simulink model "starter_model"  (R2026a)
settings: Solver=FixedStepDiscrete  StopTime=inf  FixedStep=0.01  EnableMultiTasking=on
undefined symbols (not defined in the file): dspblkCoreblockFVToolHelper, gcbh
settings Model: SILPILModeSetting=veronly  ExtModeTrigDuration=2  Creator=AdePratamaSuryoKusum  LastModifiedBy=AdePratamaSuryoKusum
settings DataIOCC: ExternalInput=milInput
settings HardwareCC: ProdBitPerInt=16.0  ProdBitPerPointer=16.0  ProdBitPerSizeT=16.0  ProdBitPerPtrDiffT=16.0  ProdWordSize=8.0  ProdHWDeviceType=Atmel->AVR
settings RTWCC: SystemTargetFile=ert.tlc  HardwareBoard=Arduino Uno  TLCOptions="-aInlineSetEventsForThisBaseRateFcn=TLC_FALSE -aSuppressMultiTaskScheduler=TLC_FALSE   -aRateBasedStepFcn=1"  Toolchain=Arduino AVR  BuildConfiguration=Faster Runs  Description=Embedded Coder
settings ERTTargetCC: ExtModeTransport=3.0  ExtModeAutomaticAllocSize=off  ExtModeStaticAllocSize=250.0  SupportContinuousTime=on  SupportVariableSizeSignals=on

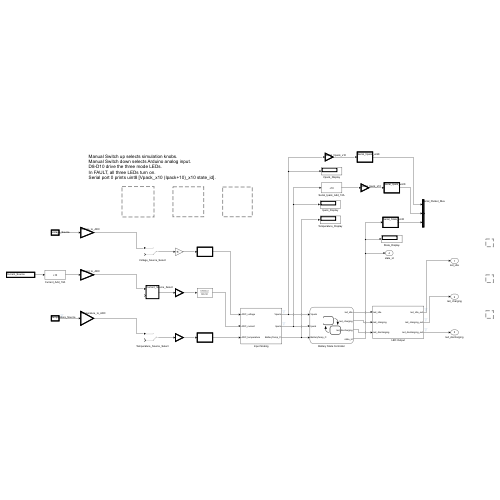
[thumbnail: Simulink's stored preview of the top-level diagram]
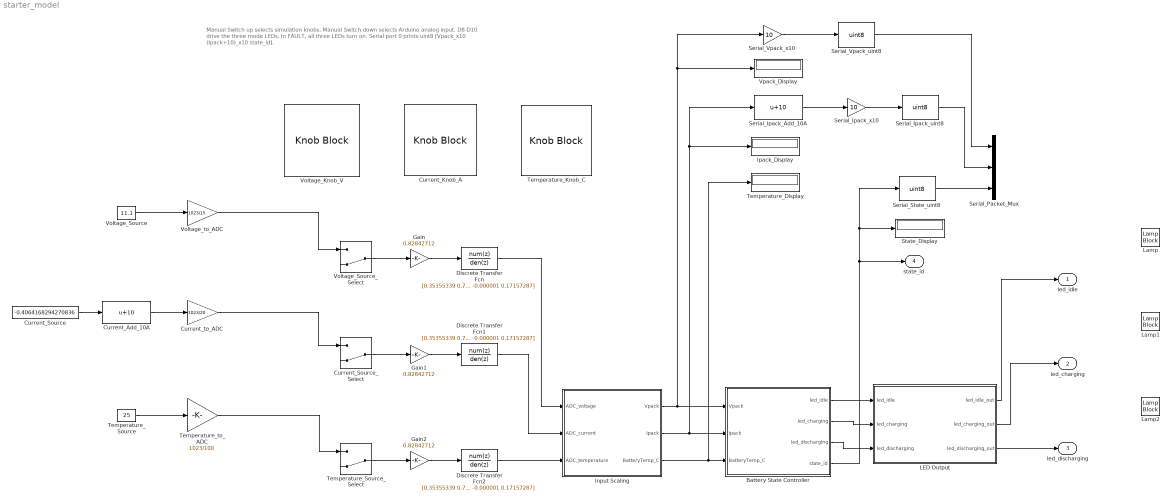
== system starter_model ==
  note: Manual Switch up selects simulation knobs.
      | Manual Switch down selects Arduino analog input.
      | D8-D10 drive the three mode LEDs.
      | In FAULT, all three LEDs turn on.
      | Serial port 0 prints uint8 [Vpack_x10 (Ipack+10)_x10 state_id].
  Battery State Controller : Stateflow chart  TreatAsAtomicUnit=on
  Current_Add_10A : Bias  Bias=10  SaturateOnIntegerOverflow=off
  Current_Knob_A : KnobBlock  ScaleMin=-10  ScaleMax=10
  Current_Source : Constant  Value=-0.4064168294270836
  Current_Source_Select : ManualSwitch  CurrentSetting=0
  Current_to_ADC : Gain  Gain=1023/20
  Discrete Transfer Fcn : DiscreteTransferFcn  LoadFcn=dspblkCoreblockFVToolHelper(gcbh,'load');  Numerator=[0.35355339 0.70710678 0.35355339]  Denominator=[1 -0.000001 0.17157287]
      settings: CopyFcn=dspblkCoreblockFVToolHelper(gcbh,'copy');  DeleteFcn=dspblkCoreblockFVToolHelper(gcbh,'close');  ModelCloseFcn=dspblkCoreblockFVToolHelper(gcbh,'close');  PreSaveFcn=dspblkCoreblockFVToolHelper(gcbh,'presave');  PostSaveFcn=dspblkCoreblockFVToolHelper(gcbh,'postsave');  CloseFcn=dspblkCoreblockFVToolHelper(gcbh,'close');
  Discrete Transfer Fcn1 : DiscreteTransferFcn  LoadFcn=dspblkCoreblockFVToolHelper(gcbh,'load');  Numerator=[0.35355339 0.70710678 0.35355339]  Denominator=[1 -0.000001 0.17157287]
      settings: CopyFcn=dspblkCoreblockFVToolHelper(gcbh,'copy');  DeleteFcn=dspblkCoreblockFVToolHelper(gcbh,'close');  ModelCloseFcn=dspblkCoreblockFVToolHelper(gcbh,'close');  PreSaveFcn=dspblkCoreblockFVToolHelper(gcbh,'presave');  PostSaveFcn=dspblkCoreblockFVToolHelper(gcbh,'postsave');  CloseFcn=dspblkCoreblockFVToolHelper(gcbh,'close');
  Discrete Transfer Fcn2 : DiscreteTransferFcn  LoadFcn=dspblkCoreblockFVToolHelper(gcbh,'load');  Numerator=[0.35355339 0.70710678 0.35355339]  Denominator=[1 -0.000001 0.17157287]
      settings: CopyFcn=dspblkCoreblockFVToolHelper(gcbh,'copy');  DeleteFcn=dspblkCoreblockFVToolHelper(gcbh,'close');  ModelCloseFcn=dspblkCoreblockFVToolHelper(gcbh,'close');  PreSaveFcn=dspblkCoreblockFVToolHelper(gcbh,'presave');  PostSaveFcn=dspblkCoreblockFVToolHelper(gcbh,'postsave');  CloseFcn=dspblkCoreblockFVToolHelper(gcbh,'close');
  Gain : Gain  Gain=0.82842712
  Gain1 : Gain  Gain=0.82842712
  Gain2 : Gain  Gain=0.82842712
  Input Scaling : Subsystem
  Ipack_Display : Display
  LED Output : Subsystem
  Lamp : LampBlock  LabelPosition=Hide  DefaultColor=[192.0, 192.0, 192.0]
  Lamp1 : LampBlock  LabelPosition=Hide  DefaultColor=[192.0, 192.0, 192.0]
  Lamp2 : LampBlock  LabelPosition=Hide  DefaultColor=[192.0, 192.0, 192.0]
  Serial_Ipack_Add_10A : Bias  Bias=10  SaturateOnIntegerOverflow=off
  Serial_Ipack_uint8 : DataTypeConversion  OutDataTypeStr=uint8  SaturateOnIntegerOverflow=off  RndMeth=Floor
  Serial_Ipack_x10 : Gain  Gain=10
  Serial_Packet_Mux : Mux  Inputs=3
  Serial_State_uint8 : DataTypeConversion  OutDataTypeStr=uint8  SaturateOnIntegerOverflow=off  RndMeth=Floor
  Serial_Vpack_uint8 : DataTypeConversion  OutDataTypeStr=uint8  SaturateOnIntegerOverflow=off  RndMeth=Floor
  Serial_Vpack_x10 : Gain  Gain=10
  State_Display : Display
  Temperature_Display : Display
  Temperature_Knob_C : KnobBlock
  Temperature_Source : Constant  Value=25
  Temperature_Source_Select : ManualSwitch  CurrentSetting=0
  Temperature_to_ADC : Gain  Gain=1023/100
  Voltage_Knob_V : KnobBlock  ScaleMax=15
  Voltage_Source : Constant  Value=11.1
  Voltage_Source_Select : ManualSwitch  CurrentSetting=0
  Voltage_to_ADC : Gain  Gain=1023/15
  Vpack_Display : Display
  led_idle : Outport
  led_charging : Outport  Port=2
  led_discharging : Outport  Port=3
  state_id : Outport  Port=4
  wires:
  Current_Add_10A/1 -> Current_to_ADC/1
  Current_Source/1 -> Current_Add_10A/1
  Input Scaling/1(Vpack) -> Battery State Controller/1(Vpack), Serial_Vpack_x10/1, Vpack_Display/1
  Voltage_to_ADC/1 -> Voltage_Source_Select/1
  Voltage_Source_Select/1 -> Gain/1
  Voltage_Source/1 -> Voltage_to_ADC/1
  Temperature_Source_Select/1 -> Gain2/1
  Temperature_Source/1 -> Temperature_to_ADC/1
  Current_to_ADC/1 -> Current_Source_Select/1
  Temperature_to_ADC/1 -> Temperature_Source_Select/1
  Current_Source_Select/1 -> Gain1/1
  Input Scaling/2(Ipack) -> Ipack_Display/1, Serial_Ipack_Add_10A/1, Battery State Controller/2(Ipack)
  Input Scaling/3(BatteryTemp_C) -> Temperature_Display/1, Battery State Controller/3(BatteryTemp_C)
  Serial_Vpack_x10/1 -> Serial_Vpack_uint8/1
  Serial_Ipack_Add_10A/1 -> Serial_Ipack_x10/1
  Battery State Controller/1(led_idle) -> LED Output/1(led_idle)
  LED Output/2(led_charging_out) -> led_charging/1
  Battery State Controller/2(led_charging) -> LED Output/2(led_charging)
  Battery State Controller/3(led_discharging) -> LED Output/3(led_discharging)
  Battery State Controller/4(state_id) -> Serial_State_uint8/1, State_Display/1, state_id/1
  Serial_Vpack_uint8/1 -> Serial_Packet_Mux/1
  Serial_State_uint8/1 -> Serial_Packet_Mux/3
  Serial_Ipack_x10/1 -> Serial_Ipack_uint8/1
  LED Output/1(led_idle_out) -> led_idle/1
  LED Output/3(led_discharging_out) -> led_discharging/1
  Serial_Ipack_uint8/1 -> Serial_Packet_Mux/2
  Discrete Transfer Fcn/1 -> Input Scaling/1(ADC_voltage)
  Discrete Transfer Fcn1/1 -> Input Scaling/2(ADC_current)
  Discrete Transfer Fcn2/1 -> Input Scaling/3(ADC_temperature)
  Gain/1 -> Discrete Transfer Fcn/1
  Gain1/1 -> Discrete Transfer Fcn1/1
  Gain2/1 -> Discrete Transfer Fcn2/1

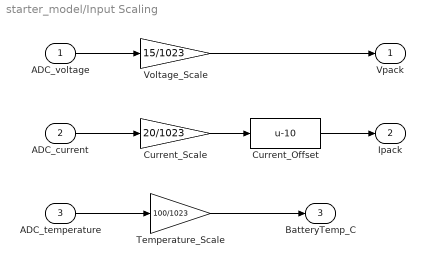
== system starter_model/Input Scaling ==
  ADC_voltage : Inport
  ADC_current : Inport  Port=2
  ADC_temperature : Inport  Port=3
  Current_Offset : Bias  Bias=-10  SaturateOnIntegerOverflow=off
  Current_Scale : Gain  Gain=20/1023
  Temperature_Scale : Gain  Gain=100/1023
  Voltage_Scale : Gain  Gain=15/1023
  Vpack : Outport
  Ipack : Outport  Port=2
  BatteryTemp_C : Outport  Port=3
  wires:
  ADC_voltage/1 -> Voltage_Scale/1
  Voltage_Scale/1 -> Vpack/1
  ADC_current/1 -> Current_Scale/1
  Current_Scale/1 -> Current_Offset/1
  Current_Offset/1 -> Ipack/1
  ADC_temperature/1 -> Temperature_Scale/1
  Temperature_Scale/1 -> BatteryTemp_C/1

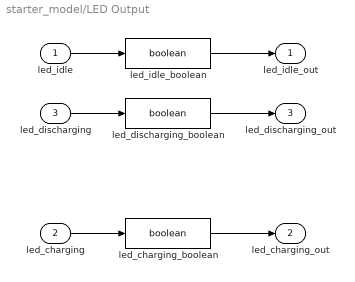
== system starter_model/LED Output ==
  led_idle : Inport
  led_charging : Inport  Port=2
  led_discharging : Inport  Port=3
  led_charging_boolean : DataTypeConversion  OutDataTypeStr=boolean  SaturateOnIntegerOverflow=off  RndMeth=Floor
  led_discharging_boolean : DataTypeConversion  OutDataTypeStr=boolean  SaturateOnIntegerOverflow=off  RndMeth=Floor
  led_idle_boolean : DataTypeConversion  OutDataTypeStr=boolean  SaturateOnIntegerOverflow=off  RndMeth=Floor
  led_idle_out : Outport
  led_charging_out : Outport  Port=2
  led_discharging_out : Outport  Port=3
  wires:
  led_charging/1 -> led_charging_boolean/1
  led_discharging/1 -> led_discharging_boolean/1
  led_idle/1 -> led_idle_boolean/1
  led_idle_boolean/1 -> led_idle_out/1
  led_discharging_boolean/1 -> led_discharging_out/1
  led_charging_boolean/1 -> led_charging_out/1

== stateflow chart starter_model/Battery State Controller ==
  data: Vpack input double; Ipack input double; led_idle output boolean; led_charging output boolean; led_discharging output boolean; state_id output uint8; BatteryTemp_C input double
